simulink model "correct_sm_circle (1)"  (R2022b)
settings: Solver=VariableStepAuto  StartTime=0.0  StopTime=25  RelTol=1e-3
values from neighbouring files (symbols this model uses):
  Fxg = 0.005    [constants (3).m]
  Fyg = 0.005    [constants (3).m]
  g = 9.81    [constants (3).m]
  Ixx = 2.3951 * 10^-5    (= 2.3951e-05)    [constants (3).m]
  Iyy = 2.3951 * 10^-5    (= 2.3951e-05)    [constants (3).m]
  Izz = 3.2347 * 10^-5    (= 3.2347e-05)    [constants (3).m]
  kf = 0.005022    [constants (3).m]
  km = 1.858*10^-5    (= 1.858e-05)    [constants (3).m]
  L = 32 * 10^-3    (= 0.032)    [constants (3).m]
  m = 0.034    [constants (3).m]
libraries: slpidlib x6, matrix_library x1, aerolibutil x1
settings Model: Creator=nayan  LastModifiedBy=Sreejeet Maity
settings SolverCC: ZeroCrossAlgorithm=Adaptive
settings DebuggingCC: IgnoredZcDiagnostic=none
settings ModelReferenceCC: EnableRefExpFcnMdlSchedulingChecks=on

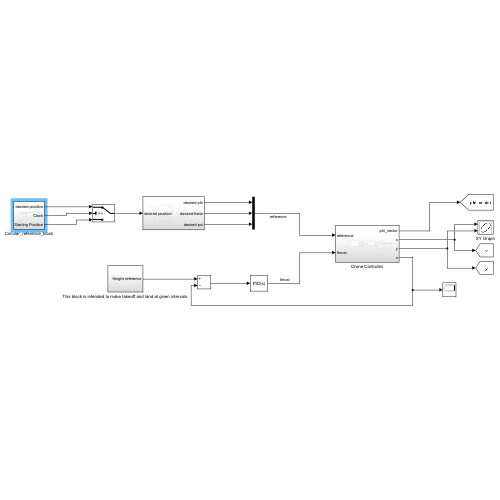
[thumbnail: Simulink's stored preview of the top-level diagram]
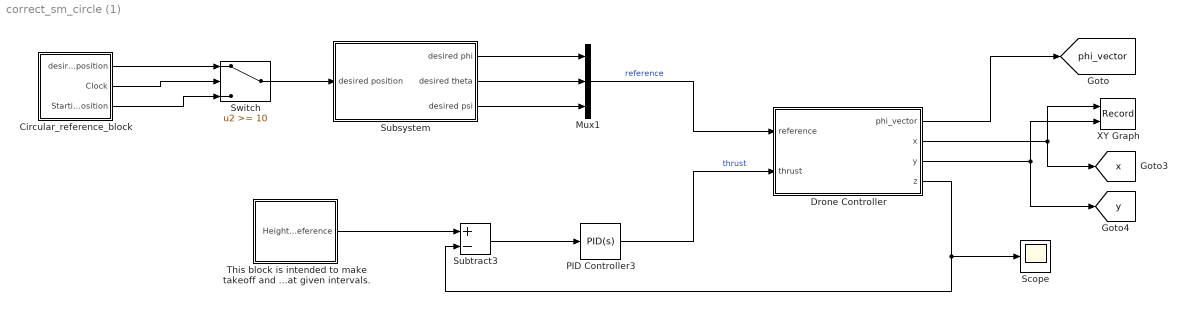
== system correct_sm_circle (1) ==
  Circular_reference_block : Subsystem
  Drone Controller : Subsystem
  Mux1 : Mux  Inputs=3
  PID Controller3 : slpidlib/PID Controller  Controller=PID  Form=Parallel  TimeDomain=Continuous-time  UseExternalTs=off  SampleTime=-1  IntegratorMethod=Forward Euler  FilterMethod=Forward Euler  ControllerParametersSource=internal  P=291  I=47.33  UseKiTs=off  D=18.69  N=1478  UseFilter=on  TunerSelectOption=Transfer Function Based (PID Tuner App)  InitialConditionSource=internal  InitialConditionForIntegrator=0  InitialConditionForFilter=0  DifferentiatorICPrevScaledInput=0  ExternalReset=none  TrackingMode=off  Kt=1  LimitOutput=off  SatLimitsSource=internal  UpperSaturationLimit=inf  LowerSaturationLimit=-inf  LinearizeAsGain=on  AntiWindupMode=none  Kb=1  LimitIntegrator=off  UpperIntegratorSaturationLimit=inf  LowerIntegratorSaturationLimit=-inf  POutMin=[]  POutMax=[]  IOutMin=[]  IOutMax=[]  DOutMin=[]  DOutMax=[]  NOutMin=[]  NOutMax=[]  SumOutMin=[]  SumOutMax=[]  SaturationOutMin=[]  SaturationOutMax=[]  PParamMin=[]  PParamMax=[]  IParamMin=[]  IParamMax=[]  DParamMin=[]  DParamMax=[]  NParamMin=[]  NParamMax=[]  KbParamMin=[]  KbParamMax=[]  KtParamMin=[]  KtParamMax=[]  KbOutMin=[]  KbOutMax=[]  KtOutMin=[]  KtOutMax=[]  IntegratorOutMin=[]  IntegratorOutMax=[]  FilterOutMin=[]  FilterOutMax=[]  SumI1OutMin=[]  SumI1OutMax=[]  SumI2OutMin=[]  SumI2OutMax=[]  SumI3OutMin=[]  SumI3OutMax=[]  SumI4OutMin=[]  SumI4OutMax=[]  SumDOutMin=[]  SumDOutMax=[]  DifferentiatorOutMin=[]  DifferentiatorOutMax=[]  FilterDiffOutCoefMin=[]  FilterDiffOutCoefMax=[]  ReciprocalOutMin=[]  ReciprocalOutMax=[]  SumDenOutMin=[]  SumDenOutMax=[]  SumNumOutMin=[]  SumNumOutMax=[]  DivideOutMin=[]  DivideOutMax=[]  UdiffTsProdOutMin=[]  UdiffTsProdOutMax=[]  NTsProdOutMin=[]  NTsProdOutMax=[]  UintegralTsProdOutMin=[]  UintegralTsProdOutMax=[]  UngainTsProdOutMin=[]  UngainTsProdOutMax=[]  ClampingZeroOutDataTypeStr=Inherit: Inherit via back propagation  ClampingZeroOutMin=[]  ClampingZeroOutMax=[]  FilterDenConstantOutDataTypeStr=Inherit: Inherit via back propagation  FilterDenConstantOutMin=[]  FilterDenConstantOutMax=[]  PCopyOutDataTypeStr=Inherit: Inherit via back propagation  PCopyOutMin=[]  PCopyOutMax=[]  NCopyOutDataTypeStr=Inherit: Inherit via back propagation  NCopyOutMin=[]  NCopyOutMax=[]  IntegratorContinuousStateAttributes=''  IntegratorStateMustResolveToSignalObject=off  IntegratorRTWStateStorageClass=Auto  FilterContinuousStateAttributes=''  FilterStateMustResolveToSignalObject=off  FilterRTWStateStorageClass=Auto  ParallelPVariant=InternalParameters  IdealPVariant=Disabled  IVariant=InternalParameters  DVariant=InternalParameters  IntegratorVariant=Continuous  SatVariant=Disabled  AWVariant=Passthrough  PCopyVariant=Disabled  TRVariant=Disabled  FdbkBlocksVariant=Forward  IdealPFdbkVariant=Disabled  SatFdbkVariant=Disabled  DerivativeFilterVariant=ContFilter  NVariant=InternalParameters  NCopyVariant=Disabled  FilterICVariant=InternalICsFilter  IntegratorICVariant=InternalICs  ExternalResetVariant=Disabled  TRSumVariant=Passthrough  SumFdbkVariant=Disabled  SumVariant=Sum_PID  TsampFilterVariant=InternalTs  TsampNgainVariant=Passthrough  TsampIntegralVariant=Passthrough  ExternalSaturationOutDataTypeStr=Inherit: Same as second input
  Scope : Scope
  Subsystem : Subsystem
  Subtract3 : Sum  Inputs=+-
  Switch : Switch  Threshold=10  SaturateOnIntegerOverflow=off  InputSameDT=off
  This block is intended to make takeoff and land at given intervals. : Subsystem
  XY Graph : Record  FileSettingsInternal="{\"entries\":[{\"content\":{\"excelSettings\":{\"content\":{},\"type\":\"Streamout.ExcelSettings\"}},\"type\":\"Streamout.FileSettingStorage\",\"uuid\":\"8c642e62-005c-4423-a761-cbdb6bbecf0f\"}],\"packageUris\":[\"http://schema.mathworks.com/mf0/streamout_blocks/R2020a\"],\"version\":\"1.0\"}"  Layout=[1 1]  SignalsInternal="{\"entries\":[{\"content\":{\"signals\":[{\"content\":{\"blockPath\":[\"correct_sm_circle/XY Graph\"],\"channel\":[],\"dimensions\":[1],\"domain\":\"correct_sm_circle/XY Graph\",\"lineColor\":\"#a2142f\",\"plots\":[1],\"port\":1,\"sid\":[\"\"],\"signalID\":12972,\"signalName\":\"Drone Controller:2\"},\"type\":\"RecordBlkView.Signal\",\"uuid\":\"ff125678-109d-4bf1-ad2c-892bd237ab7f\"},{\"content\":{\"blockPath\":[\"correct_sm_circle/XY Graph\"],\"channel\":[],\"dimensions\":[1],\"domain\":\"correct_sm_circle/XY Graph\",\"lineColor\":\"#139fff\",\"plots\":[1],\"port\":2,\"sid\":[\"\"],\"signalID\":12976,\"signalName\":\"Drone Controller:3\"},\"type\":\"RecordBlkView.Signal\",\"uuid\":\"d1c5deef-ede5-4cd3-9f15-060bb912ac46\"}]},\"type\":\"RecordBlkView.InputSignals\",\"uuid\":\"1252a0e8-627c-4691-9929-d6fd4d200b48\"}],\"packageUris\":[\"http://schema.mathworks.com/mf0/streamout_blocks/R2020a\"],\"version\":\"1.0\"}"  VisualizationBindings="{\"xyplotplugin\":{\"info\":[{\"series\":[{\"bindingParametersList\":[{\"parameter\":\"X-Axis\",\"signalID\":12972,\"signalName\":\"Drone Controller:2\"},{\"parameter\":\"Y-Axis\",\"signalID\":12976,\"signalName\":\"Drone Controller:3\"}],\"seriesID\":36752}],\"subplotID\":1}]}}"  CompatibilityTag=XY
  tag scope: phi_vector=global, x=global, y=global
  wires:
  Subtract3/1 -> PID Controller3/1
  Subsystem/1(desired phi) -> Mux1/1
  Subsystem/2(desired theta) -> Mux1/2
  Subsystem/3(desired psi) -> Mux1/3
  Switch/1 -> Subsystem/1(desired position)
  Circular_reference_block/1(desired position) -> Switch/1
  Circular_reference_block/2(Clock) -> Switch/2
  Circular_reference_block/3(Starting Position) -> Switch/3
  This block is intended to make takeoff and land at given intervals./1(Height reference) -> Subtract3/1
  Drone Controller/2(x) -> XY Graph/1, [x]
  Drone Controller/3(y) -> XY Graph/2, [y]
  Drone Controller/4(z) -> Subtract3/2, Scope/1
  Mux1/1 -> Drone Controller/1(reference)  "reference"
  PID Controller3/1 -> Drone Controller/2(thrust)  "thrust"
  Drone Controller/1(phi_vector) -> [phi_vector]

== system correct_sm_circle (1)/Circular_reference_block ==
  Circular_reference : Subsystem
  Desired Position : Scope
  Initial Position : Constant  Value=[1 ; 0]
  Mux3 : Mux  Inputs=2
  desired position : Outport
  Clock : Outport  Port=2
  Starting Position : Outport  Port=3
  wires:
  Initial Position/1 -> Starting Position/1
  Mux3/1 -> desired position/1, Desired Position/1  "desired position"
  Circular_reference/2(cos(t-10)) -> Mux3/1
  Circular_reference/3(sin(t-10)) -> Mux3/2
  Circular_reference/1(Clock) -> Clock/1

== system correct_sm_circle (1)/Drone Controller ==
  reference : Inport
  thrust : Inport  Port=2
  Attitude Controller : Subsystem
  Drone_1 : Subsystem
  Mux : Mux
  phi_vector : Outport
  x : Outport  Port=2
  y : Outport  Port=3
  z : Outport  Port=4
  wires:
  Drone_1/4(z) -> z/1
  Attitude Controller/1(w1_square) -> Mux/1
  Attitude Controller/3(w3_square) -> Mux/3
  Drone_1/2(x) -> x/1
  Mux/1 -> Drone_1/1(squares of motor omega in rpm)  "squares of motor omega in rpm"
  Drone_1/3(y) -> y/1
  Attitude Controller/2(w2_square) -> Mux/2
  Attitude Controller/4(w4_square) -> Mux/4
  Drone_1/1(phi_vector) -> phi_vector/1
  thrust/1 -> Attitude Controller/2("thrust ")
  reference/1 -> Attitude Controller/1(roll pitch yaw reference)

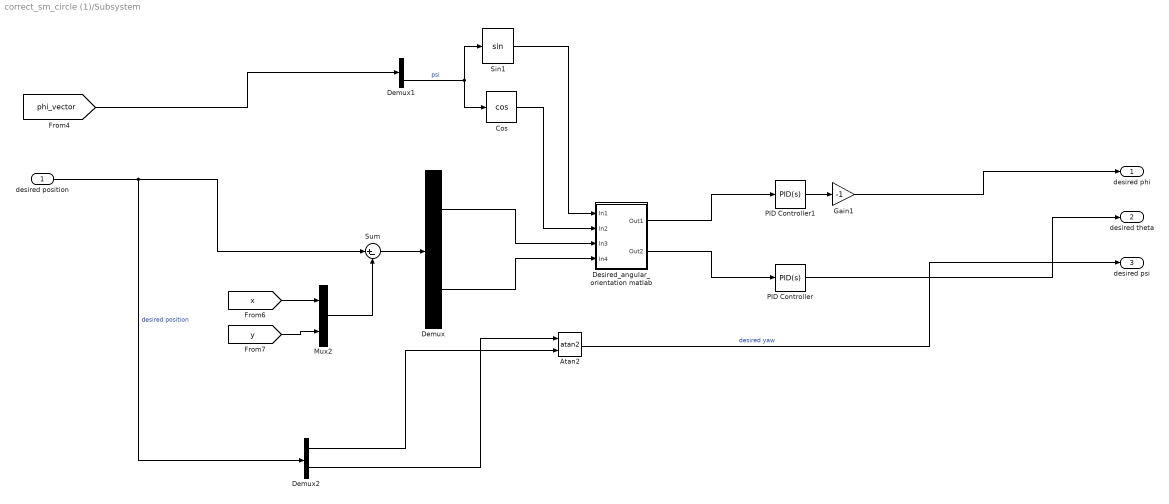
== system correct_sm_circle (1)/Subsystem ==
  desired position : Inport
  Atan2 : Trigonometry  Operator=atan2
  Cos : Trigonometry  Operator=cos
  Demux : Demux  Outputs=2
  Demux1 : Demux  Outputs=3
  Demux2 : Demux  Outputs=2
  Desired_angular_orientation matlab : Subsystem
  Gain1 : Gain  Gain=-1
  Mux2 : Mux  Inputs=2
  PID Controller : slpidlib/PID Controller  Controller=PID  Form=Parallel  TimeDomain=Continuous-time  UseExternalTs=off  SampleTime=-1  IntegratorMethod=Forward Euler  FilterMethod=Forward Euler  ControllerParametersSource=internal  P=0.43  I=0.043  UseKiTs=off  D=0.042  N=10000  UseFilter=on  TunerSelectOption=Transfer Function Based (PID Tuner App)  InitialConditionSource=internal  InitialConditionForIntegrator=0  InitialConditionForFilter=0  DifferentiatorICPrevScaledInput=0  ExternalReset=none  TrackingMode=off  Kt=1  LimitOutput=off  SatLimitsSource=internal  UpperSaturationLimit=inf  LowerSaturationLimit=-inf  LinearizeAsGain=on  AntiWindupMode=none  Kb=1  LimitIntegrator=off  UpperIntegratorSaturationLimit=inf  LowerIntegratorSaturationLimit=-inf  POutMin=[]  POutMax=[]  IOutMin=[]  IOutMax=[]  DOutMin=[]  DOutMax=[]  NOutMin=[]  NOutMax=[]  SumOutMin=[]  SumOutMax=[]  SaturationOutMin=[]  SaturationOutMax=[]  PParamMin=[]  PParamMax=[]  IParamMin=[]  IParamMax=[]  DParamMin=[]  DParamMax=[]  NParamMin=[]  NParamMax=[]  KbParamMin=[]  KbParamMax=[]  KtParamMin=[]  KtParamMax=[]  KbOutMin=[]  KbOutMax=[]  KtOutMin=[]  KtOutMax=[]  IntegratorOutMin=[]  IntegratorOutMax=[]  FilterOutMin=[]  FilterOutMax=[]  SumI1OutMin=[]  SumI1OutMax=[]  SumI2OutMin=[]  SumI2OutMax=[]  SumI3OutMin=[]  SumI3OutMax=[]  SumI4OutMin=[]  SumI4OutMax=[]  SumDOutMin=[]  SumDOutMax=[]  DifferentiatorOutMin=[]  DifferentiatorOutMax=[]  FilterDiffOutCoefMin=[]  FilterDiffOutCoefMax=[]  ReciprocalOutMin=[]  ReciprocalOutMax=[]  SumDenOutMin=[]  SumDenOutMax=[]  SumNumOutMin=[]  SumNumOutMax=[]  DivideOutMin=[]  DivideOutMax=[]  UdiffTsProdOutMin=[]  UdiffTsProdOutMax=[]  NTsProdOutMin=[]  NTsProdOutMax=[]  UintegralTsProdOutMin=[]  UintegralTsProdOutMax=[]  UngainTsProdOutMin=[]  UngainTsProdOutMax=[]  ClampingZeroOutDataTypeStr=Inherit: Inherit via back propagation  ClampingZeroOutMin=[]  ClampingZeroOutMax=[]  FilterDenConstantOutDataTypeStr=Inherit: Inherit via back propagation  FilterDenConstantOutMin=[]  FilterDenConstantOutMax=[]  PCopyOutDataTypeStr=Inherit: Inherit via back propagation  PCopyOutMin=[]  PCopyOutMax=[]  NCopyOutDataTypeStr=Inherit: Inherit via back propagation  NCopyOutMin=[]  NCopyOutMax=[]  IntegratorContinuousStateAttributes=''  IntegratorStateMustResolveToSignalObject=off  IntegratorRTWStateStorageClass=Auto  FilterContinuousStateAttributes=''  FilterStateMustResolveToSignalObject=off  FilterRTWStateStorageClass=Auto  ParallelPVariant=InternalParameters  IdealPVariant=Disabled  IVariant=InternalParameters  DVariant=InternalParameters  IntegratorVariant=Continuous  SatVariant=Disabled  AWVariant=Passthrough  PCopyVariant=Disabled  TRVariant=Disabled  FdbkBlocksVariant=Forward  IdealPFdbkVariant=Disabled  SatFdbkVariant=Disabled  DerivativeFilterVariant=ContFilter  NVariant=InternalParameters  NCopyVariant=Disabled  FilterICVariant=InternalICsFilter  IntegratorICVariant=InternalICs  ExternalResetVariant=Disabled  TRSumVariant=Passthrough  SumFdbkVariant=Disabled  SumVariant=Sum_PID  TsampFilterVariant=InternalTs  TsampNgainVariant=Passthrough  TsampIntegralVariant=Passthrough  ExternalSaturationOutDataTypeStr=Inherit: Same as second input
  PID Controller1 : slpidlib/PID Controller  Controller=PID  Form=Parallel  TimeDomain=Continuous-time  UseExternalTs=off  SampleTime=-1  IntegratorMethod=Forward Euler  FilterMethod=Forward Euler  ControllerParametersSource=internal  P=0.43  I=0.0412  UseKiTs=off  D=0.043  N=10000  UseFilter=on  TunerSelectOption=Transfer Function Based (PID Tuner App)  InitialConditionSource=internal  InitialConditionForIntegrator=0  InitialConditionForFilter=0  DifferentiatorICPrevScaledInput=0  ExternalReset=none  TrackingMode=off  Kt=1  LimitOutput=off  SatLimitsSource=internal  UpperSaturationLimit=inf  LowerSaturationLimit=-inf  LinearizeAsGain=on  AntiWindupMode=none  Kb=1  LimitIntegrator=off  UpperIntegratorSaturationLimit=inf  LowerIntegratorSaturationLimit=-inf  POutMin=[]  POutMax=[]  IOutMin=[]  IOutMax=[]  DOutMin=[]  DOutMax=[]  NOutMin=[]  NOutMax=[]  SumOutMin=[]  SumOutMax=[]  SaturationOutMin=[]  SaturationOutMax=[]  PParamMin=[]  PParamMax=[]  IParamMin=[]  IParamMax=[]  DParamMin=[]  DParamMax=[]  NParamMin=[]  NParamMax=[]  KbParamMin=[]  KbParamMax=[]  KtParamMin=[]  KtParamMax=[]  KbOutMin=[]  KbOutMax=[]  KtOutMin=[]  KtOutMax=[]  IntegratorOutMin=[]  IntegratorOutMax=[]  FilterOutMin=[]  FilterOutMax=[]  SumI1OutMin=[]  SumI1OutMax=[]  SumI2OutMin=[]  SumI2OutMax=[]  SumI3OutMin=[]  SumI3OutMax=[]  SumI4OutMin=[]  SumI4OutMax=[]  SumDOutMin=[]  SumDOutMax=[]  DifferentiatorOutMin=[]  DifferentiatorOutMax=[]  FilterDiffOutCoefMin=[]  FilterDiffOutCoefMax=[]  ReciprocalOutMin=[]  ReciprocalOutMax=[]  SumDenOutMin=[]  SumDenOutMax=[]  SumNumOutMin=[]  SumNumOutMax=[]  DivideOutMin=[]  DivideOutMax=[]  UdiffTsProdOutMin=[]  UdiffTsProdOutMax=[]  NTsProdOutMin=[]  NTsProdOutMax=[]  UintegralTsProdOutMin=[]  UintegralTsProdOutMax=[]  UngainTsProdOutMin=[]  UngainTsProdOutMax=[]  ClampingZeroOutDataTypeStr=Inherit: Inherit via back propagation  ClampingZeroOutMin=[]  ClampingZeroOutMax=[]  FilterDenConstantOutDataTypeStr=Inherit: Inherit via back propagation  FilterDenConstantOutMin=[]  FilterDenConstantOutMax=[]  PCopyOutDataTypeStr=Inherit: Inherit via back propagation  PCopyOutMin=[]  PCopyOutMax=[]  NCopyOutDataTypeStr=Inherit: Inherit via back propagation  NCopyOutMin=[]  NCopyOutMax=[]  IntegratorContinuousStateAttributes=''  IntegratorStateMustResolveToSignalObject=off  IntegratorRTWStateStorageClass=Auto  FilterContinuousStateAttributes=''  FilterStateMustResolveToSignalObject=off  FilterRTWStateStorageClass=Auto  ParallelPVariant=InternalParameters  IdealPVariant=Disabled  IVariant=InternalParameters  DVariant=InternalParameters  IntegratorVariant=Continuous  SatVariant=Disabled  AWVariant=Passthrough  PCopyVariant=Disabled  TRVariant=Disabled  FdbkBlocksVariant=Forward  IdealPFdbkVariant=Disabled  SatFdbkVariant=Disabled  DerivativeFilterVariant=ContFilter  NVariant=InternalParameters  NCopyVariant=Disabled  FilterICVariant=InternalICsFilter  IntegratorICVariant=InternalICs  ExternalResetVariant=Disabled  TRSumVariant=Passthrough  SumFdbkVariant=Disabled  SumVariant=Sum_PID  TsampFilterVariant=InternalTs  TsampNgainVariant=Passthrough  TsampIntegralVariant=Passthrough  ExternalSaturationOutDataTypeStr=Inherit: Same as second input
  Sin1 : Trigonometry
  Sum : Sum  Inputs=|+-
  desired phi : Outport
  desired theta : Outport  Port=2
  desired psi : Outport  Port=3
  wires:
  Sum/1 -> Demux/1
  PID Controller/1 -> desired theta/1
  PID Controller1/1 -> Gain1/1
  Gain1/1 -> desired phi/1
  Demux1/3 -> Cos/1, Sin1/1  "psi"
  [x] -> Mux2/1
  Mux2/1 -> Sum/2
  [y] -> Mux2/2
  [phi_vector] -> Demux1/1
  desired position/1 -> Demux2/1, Sum/1  "desired position"
  Atan2/1 -> desired psi/1  "desired yaw"
  Demux2/2 -> Atan2/1
  Demux2/1 -> Atan2/2
  Sin1/1 -> Desired_angular_orientation matlab/1(In1)
  Cos/1 -> Desired_angular_orientation matlab/2(In2)
  Demux/1 -> Desired_angular_orientation matlab/3(In3)
  Demux/2 -> Desired_angular_orientation matlab/4(In4)
  Desired_angular_orientation matlab/1(Out1) -> PID Controller1/1
  Desired_angular_orientation matlab/2(Out2) -> PID Controller/1

== system correct_sm_circle (1)/This block is intended to make takeoff and land at given intervals. ==
  Clock : Clock
  Constant : Constant
  Constant3 : Constant  Value=0
  Switch1 : Switch  Threshold=20  SaturateOnIntegerOverflow=off  InputSameDT=off
  Height reference : Outport
  wires:
  Clock/1 -> Switch1/2
  Constant/1 -> Switch1/3  "Height reference"
  Constant3/1 -> Switch1/1  "Height reference"
  Switch1/1 -> Height reference/1  "Height reference"

== system correct_sm_circle (1)/Circular_reference_block/Circular_reference ==
  Clock1 : Clock
  Cos : Trigonometry  Operator=cos
  Sin1 : Trigonometry
  Subtract : Sum  Inputs=+-
  time to take_off : Constant  Value=10
  Clock : Outport
  cos(t-10) : Outport  Port=2
  sin(t-10) : Outport  Port=3
  wires:
  Subtract/1 -> Cos/1, Sin1/1
  Clock1/1 -> Clock/1, Subtract/1
  Cos/1 -> cos(t-10)/1
  time to take_off/1 -> Subtract/2
  Sin1/1 -> sin(t-10)/1

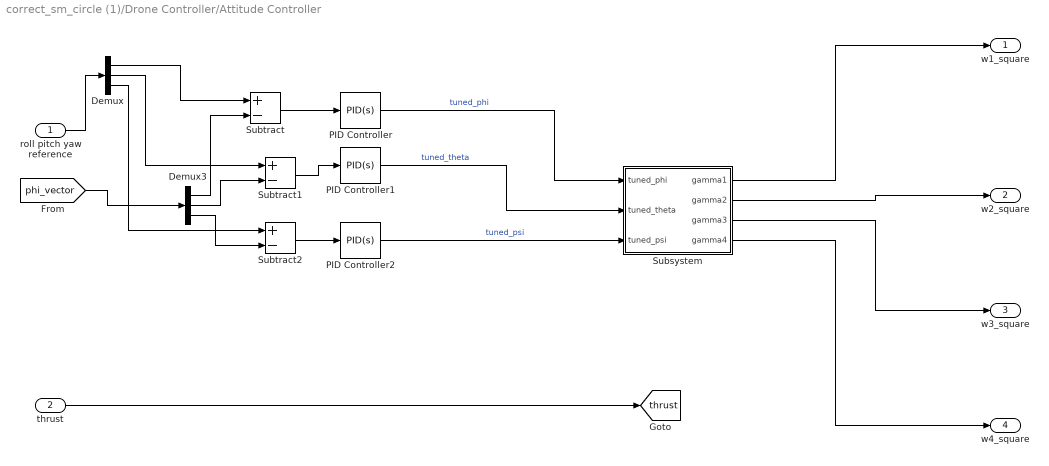
== system correct_sm_circle (1)/Drone Controller/Attitude Controller ==
  roll pitch yaw reference : Inport
  "thrust " : Inport  Port=2
  Demux : Demux  Outputs=3
  Demux3 : Demux  Outputs=3
  PID Controller : slpidlib/PID Controller  Controller=PID  Form=Parallel  TimeDomain=Continuous-time  UseExternalTs=off  SampleTime=-1  IntegratorMethod=Forward Euler  FilterMethod=Forward Euler  ControllerParametersSource=internal  P=96.35  I=143.26  UseKiTs=off  D=23.32  N=10000  UseFilter=on  TunerSelectOption=Transfer Function Based (PID Tuner App)  InitialConditionSource=internal  InitialConditionForIntegrator=0  InitialConditionForFilter=0  DifferentiatorICPrevScaledInput=0  ExternalReset=none  TrackingMode=off  Kt=1  LimitOutput=off  SatLimitsSource=internal  UpperSaturationLimit=inf  LowerSaturationLimit=-inf  LinearizeAsGain=on  AntiWindupMode=none  Kb=1  LimitIntegrator=off  UpperIntegratorSaturationLimit=inf  LowerIntegratorSaturationLimit=-inf  POutMin=[]  POutMax=[]  IOutMin=[]  IOutMax=[]  DOutMin=[]  DOutMax=[]  NOutMin=[]  NOutMax=[]  SumOutMin=[]  SumOutMax=[]  SaturationOutMin=[]  SaturationOutMax=[]  PParamMin=[]  PParamMax=[]  IParamMin=[]  IParamMax=[]  DParamMin=[]  DParamMax=[]  NParamMin=[]  NParamMax=[]  KbParamMin=[]  KbParamMax=[]  KtParamMin=[]  KtParamMax=[]  KbOutMin=[]  KbOutMax=[]  KtOutMin=[]  KtOutMax=[]  IntegratorOutMin=[]  IntegratorOutMax=[]  FilterOutMin=[]  FilterOutMax=[]  SumI1OutMin=[]  SumI1OutMax=[]  SumI2OutMin=[]  SumI2OutMax=[]  SumI3OutMin=[]  SumI3OutMax=[]  SumI4OutMin=[]  SumI4OutMax=[]  SumDOutMin=[]  SumDOutMax=[]  DifferentiatorOutMin=[]  DifferentiatorOutMax=[]  FilterDiffOutCoefMin=[]  FilterDiffOutCoefMax=[]  ReciprocalOutMin=[]  ReciprocalOutMax=[]  SumDenOutMin=[]  SumDenOutMax=[]  SumNumOutMin=[]  SumNumOutMax=[]  DivideOutMin=[]  DivideOutMax=[]  UdiffTsProdOutMin=[]  UdiffTsProdOutMax=[]  NTsProdOutMin=[]  NTsProdOutMax=[]  UintegralTsProdOutMin=[]  UintegralTsProdOutMax=[]  UngainTsProdOutMin=[]  UngainTsProdOutMax=[]  ClampingZeroOutDataTypeStr=Inherit: Inherit via back propagation  ClampingZeroOutMin=[]  ClampingZeroOutMax=[]  FilterDenConstantOutDataTypeStr=Inherit: Inherit via back propagation  FilterDenConstantOutMin=[]  FilterDenConstantOutMax=[]  PCopyOutDataTypeStr=Inherit: Inherit via back propagation  PCopyOutMin=[]  PCopyOutMax=[]  NCopyOutDataTypeStr=Inherit: Inherit via back propagation  NCopyOutMin=[]  NCopyOutMax=[]  IntegratorContinuousStateAttributes=''  IntegratorStateMustResolveToSignalObject=off  IntegratorRTWStateStorageClass=Auto  FilterContinuousStateAttributes=''  FilterStateMustResolveToSignalObject=off  FilterRTWStateStorageClass=Auto  ParallelPVariant=InternalParameters  IdealPVariant=Disabled  IVariant=InternalParameters  DVariant=InternalParameters  IntegratorVariant=Continuous  SatVariant=Disabled  AWVariant=Passthrough  PCopyVariant=Disabled  TRVariant=Disabled  FdbkBlocksVariant=Forward  IdealPFdbkVariant=Disabled  SatFdbkVariant=Disabled  DerivativeFilterVariant=ContFilter  NVariant=InternalParameters  NCopyVariant=Disabled  FilterICVariant=InternalICsFilter  IntegratorICVariant=InternalICs  ExternalResetVariant=Disabled  TRSumVariant=Passthrough  SumFdbkVariant=Disabled  SumVariant=Sum_PID  TsampFilterVariant=InternalTs  TsampNgainVariant=Passthrough  TsampIntegralVariant=Passthrough  ExternalSaturationOutDataTypeStr=Inherit: Same as second input
  PID Controller1 : slpidlib/PID Controller  Controller=PID  Form=Parallel  TimeDomain=Continuous-time  UseExternalTs=off  SampleTime=-1  IntegratorMethod=Forward Euler  FilterMethod=Forward Euler  ControllerParametersSource=internal  P=96.36  I=143.5  UseKiTs=off  D=22.32  N=10000  UseFilter=on  TunerSelectOption=Transfer Function Based (PID Tuner App)  InitialConditionSource=internal  InitialConditionForIntegrator=0  InitialConditionForFilter=0  DifferentiatorICPrevScaledInput=0  ExternalReset=none  TrackingMode=off  Kt=1  LimitOutput=off  SatLimitsSource=internal  UpperSaturationLimit=inf  LowerSaturationLimit=-inf  LinearizeAsGain=on  AntiWindupMode=none  Kb=1  LimitIntegrator=off  UpperIntegratorSaturationLimit=inf  LowerIntegratorSaturationLimit=-inf  POutMin=[]  POutMax=[]  IOutMin=[]  IOutMax=[]  DOutMin=[]  DOutMax=[]  NOutMin=[]  NOutMax=[]  SumOutMin=[]  SumOutMax=[]  SaturationOutMin=[]  SaturationOutMax=[]  PParamMin=[]  PParamMax=[]  IParamMin=[]  IParamMax=[]  DParamMin=[]  DParamMax=[]  NParamMin=[]  NParamMax=[]  KbParamMin=[]  KbParamMax=[]  KtParamMin=[]  KtParamMax=[]  KbOutMin=[]  KbOutMax=[]  KtOutMin=[]  KtOutMax=[]  IntegratorOutMin=[]  IntegratorOutMax=[]  FilterOutMin=[]  FilterOutMax=[]  SumI1OutMin=[]  SumI1OutMax=[]  SumI2OutMin=[]  SumI2OutMax=[]  SumI3OutMin=[]  SumI3OutMax=[]  SumI4OutMin=[]  SumI4OutMax=[]  SumDOutMin=[]  SumDOutMax=[]  DifferentiatorOutMin=[]  DifferentiatorOutMax=[]  FilterDiffOutCoefMin=[]  FilterDiffOutCoefMax=[]  ReciprocalOutMin=[]  ReciprocalOutMax=[]  SumDenOutMin=[]  SumDenOutMax=[]  SumNumOutMin=[]  SumNumOutMax=[]  DivideOutMin=[]  DivideOutMax=[]  UdiffTsProdOutMin=[]  UdiffTsProdOutMax=[]  NTsProdOutMin=[]  NTsProdOutMax=[]  UintegralTsProdOutMin=[]  UintegralTsProdOutMax=[]  UngainTsProdOutMin=[]  UngainTsProdOutMax=[]  ClampingZeroOutDataTypeStr=Inherit: Inherit via back propagation  ClampingZeroOutMin=[]  ClampingZeroOutMax=[]  FilterDenConstantOutDataTypeStr=Inherit: Inherit via back propagation  FilterDenConstantOutMin=[]  FilterDenConstantOutMax=[]  PCopyOutDataTypeStr=Inherit: Inherit via back propagation  PCopyOutMin=[]  PCopyOutMax=[]  NCopyOutDataTypeStr=Inherit: Inherit via back propagation  NCopyOutMin=[]  NCopyOutMax=[]  IntegratorContinuousStateAttributes=''  IntegratorStateMustResolveToSignalObject=off  IntegratorRTWStateStorageClass=Auto  FilterContinuousStateAttributes=''  FilterStateMustResolveToSignalObject=off  FilterRTWStateStorageClass=Auto  ParallelPVariant=InternalParameters  IdealPVariant=Disabled  IVariant=InternalParameters  DVariant=InternalParameters  IntegratorVariant=Continuous  SatVariant=Disabled  AWVariant=Passthrough  PCopyVariant=Disabled  TRVariant=Disabled  FdbkBlocksVariant=Forward  IdealPFdbkVariant=Disabled  SatFdbkVariant=Disabled  DerivativeFilterVariant=ContFilter  NVariant=InternalParameters  NCopyVariant=Disabled  FilterICVariant=InternalICsFilter  IntegratorICVariant=InternalICs  ExternalResetVariant=Disabled  TRSumVariant=Passthrough  SumFdbkVariant=Disabled  SumVariant=Sum_PID  TsampFilterVariant=InternalTs  TsampNgainVariant=Passthrough  TsampIntegralVariant=Passthrough  ExternalSaturationOutDataTypeStr=Inherit: Same as second input
  PID Controller2 : slpidlib/PID Controller  Controller=PID  Form=Parallel  TimeDomain=Continuous-time  UseExternalTs=off  SampleTime=-1  IntegratorMethod=Forward Euler  FilterMethod=Forward Euler  ControllerParametersSource=internal  P=96.36  I=146.25  UseKiTs=off  D=22.37  N=10000  UseFilter=on  TunerSelectOption=Transfer Function Based (PID Tuner App)  InitialConditionSource=internal  InitialConditionForIntegrator=0  InitialConditionForFilter=0  DifferentiatorICPrevScaledInput=0  ExternalReset=none  TrackingMode=off  Kt=1  LimitOutput=off  SatLimitsSource=internal  UpperSaturationLimit=inf  LowerSaturationLimit=-inf  LinearizeAsGain=on  AntiWindupMode=none  Kb=1  LimitIntegrator=off  UpperIntegratorSaturationLimit=inf  LowerIntegratorSaturationLimit=-inf  POutMin=[]  POutMax=[]  IOutMin=[]  IOutMax=[]  DOutMin=[]  DOutMax=[]  NOutMin=[]  NOutMax=[]  SumOutMin=[]  SumOutMax=[]  SaturationOutMin=[]  SaturationOutMax=[]  PParamMin=[]  PParamMax=[]  IParamMin=[]  IParamMax=[]  DParamMin=[]  DParamMax=[]  NParamMin=[]  NParamMax=[]  KbParamMin=[]  KbParamMax=[]  KtParamMin=[]  KtParamMax=[]  KbOutMin=[]  KbOutMax=[]  KtOutMin=[]  KtOutMax=[]  IntegratorOutMin=[]  IntegratorOutMax=[]  FilterOutMin=[]  FilterOutMax=[]  SumI1OutMin=[]  SumI1OutMax=[]  SumI2OutMin=[]  SumI2OutMax=[]  SumI3OutMin=[]  SumI3OutMax=[]  SumI4OutMin=[]  SumI4OutMax=[]  SumDOutMin=[]  SumDOutMax=[]  DifferentiatorOutMin=[]  DifferentiatorOutMax=[]  FilterDiffOutCoefMin=[]  FilterDiffOutCoefMax=[]  ReciprocalOutMin=[]  ReciprocalOutMax=[]  SumDenOutMin=[]  SumDenOutMax=[]  SumNumOutMin=[]  SumNumOutMax=[]  DivideOutMin=[]  DivideOutMax=[]  UdiffTsProdOutMin=[]  UdiffTsProdOutMax=[]  NTsProdOutMin=[]  NTsProdOutMax=[]  UintegralTsProdOutMin=[]  UintegralTsProdOutMax=[]  UngainTsProdOutMin=[]  UngainTsProdOutMax=[]  ClampingZeroOutDataTypeStr=Inherit: Inherit via back propagation  ClampingZeroOutMin=[]  ClampingZeroOutMax=[]  FilterDenConstantOutDataTypeStr=Inherit: Inherit via back propagation  FilterDenConstantOutMin=[]  FilterDenConstantOutMax=[]  PCopyOutDataTypeStr=Inherit: Inherit via back propagation  PCopyOutMin=[]  PCopyOutMax=[]  NCopyOutDataTypeStr=Inherit: Inherit via back propagation  NCopyOutMin=[]  NCopyOutMax=[]  IntegratorContinuousStateAttributes=''  IntegratorStateMustResolveToSignalObject=off  IntegratorRTWStateStorageClass=Auto  FilterContinuousStateAttributes=''  FilterStateMustResolveToSignalObject=off  FilterRTWStateStorageClass=Auto  ParallelPVariant=InternalParameters  IdealPVariant=Disabled  IVariant=InternalParameters  DVariant=InternalParameters  IntegratorVariant=Continuous  SatVariant=Disabled  AWVariant=Passthrough  PCopyVariant=Disabled  TRVariant=Disabled  FdbkBlocksVariant=Forward  IdealPFdbkVariant=Disabled  SatFdbkVariant=Disabled  DerivativeFilterVariant=ContFilter  NVariant=InternalParameters  NCopyVariant=Disabled  FilterICVariant=InternalICsFilter  IntegratorICVariant=InternalICs  ExternalResetVariant=Disabled  TRSumVariant=Passthrough  SumFdbkVariant=Disabled  SumVariant=Sum_PID  TsampFilterVariant=InternalTs  TsampNgainVariant=Passthrough  TsampIntegralVariant=Passthrough  ExternalSaturationOutDataTypeStr=Inherit: Same as second input
  Subsystem : Subsystem
  Subtract : Sum  Inputs=+-
  Subtract1 : Sum  Inputs=+-
  Subtract2 : Sum  Inputs=+-
  w1_square : Outport
  w2_square : Outport  Port=2
  w3_square : Outport  Port=3
  w4_square : Outport  Port=4
  tag scope: thrust=global
  wires:
  Subtract2/1 -> PID Controller2/1
  Demux3/2 -> Subtract1/2
  [phi_vector] -> Demux3/1
  Demux3/3 -> Subtract2/2
  Subtract1/1 -> PID Controller1/1
  Subtract/1 -> PID Controller/1
  Demux3/1 -> Subtract/2
  roll pitch yaw reference/1 -> Demux/1
  Demux/1 -> Subtract/1
  Demux/2 -> Subtract1/1
  Demux/3 -> Subtract2/1
  "thrust "/1 -> [thrust]
  PID Controller/1 -> Subsystem/1(tuned_phi)  "tuned_phi"
  PID Controller1/1 -> Subsystem/2(tuned_theta)  "tuned_theta"
  PID Controller2/1 -> Subsystem/3(tuned_psi)  "tuned_psi"
  Subsystem/1(gamma1) -> w1_square/1
  Subsystem/2(gamma2) -> w2_square/1
  Subsystem/3(gamma3) -> w3_square/1
  Subsystem/4(gamma4) -> w4_square/1

== system correct_sm_circle (1)/Drone Controller/Drone_1 ==
  squares of motor omega in rpm : Inport
  Drone position dynamics : Subsystem
  MMA : Subsystem
  phi_vector : Outport
  x : Outport  Port=2
  y : Outport  Port=3
  z : Outport  Port=4
  wires:
  MMA/2("[Taux;Tauy;Tauz]") -> Drone position dynamics/2(tau_vector)
  MMA/1(Thrust) -> Drone position dynamics/1(thrust)
  Drone position dynamics/1(phi_vector) -> phi_vector/1
  Drone position dynamics/3(y) -> y/1
  Drone position dynamics/4(z) -> z/1
  squares of motor omega in rpm/1 -> MMA/1(w_squares_vector)
  Drone position dynamics/2(x) -> x/1

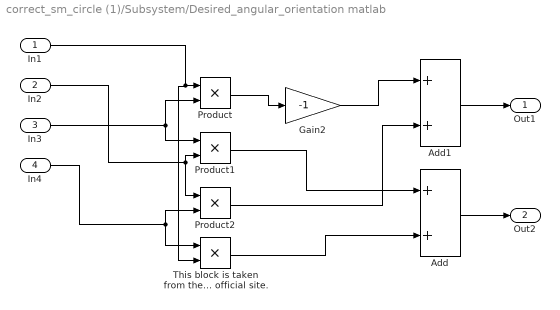
== system correct_sm_circle (1)/Subsystem/Desired_angular_orientation matlab ==
  In1 : Inport
  In2 : Inport  Port=2
  In3 : Inport  Port=3
  In4 : Inport  Port=4
  Add : Sum
  Add1 : Sum
  Gain2 : Gain  Gain=-1
  Product : Product
  Product1 : Product
  Product2 : Product
  This block is taken from the X-rotor quadrotor reference example at Matlab official site. : Product
  Out1 : Outport
  Out2 : Outport  Port=2
  wires:
  Product/1 -> Gain2/1
  Product1/1 -> Add/1
  In2/1 -> Product2/1, Product1/2
  This block is taken from the X-rotor quadrotor reference example at Matlab official site./1 -> Add/2
  In3/1 -> Product1/1, Product/2
  In4/1 -> This block is taken from the X-rotor quadrotor reference example at Matlab official site./1, Product2/2
  Product2/1 -> Add1/2
  Gain2/1 -> Add1/1
  In1/1 -> This block is taken from the X-rotor quadrotor reference example at Matlab official site./2, Product/1
  Add1/1 -> Out1/1
  Add/1 -> Out2/1

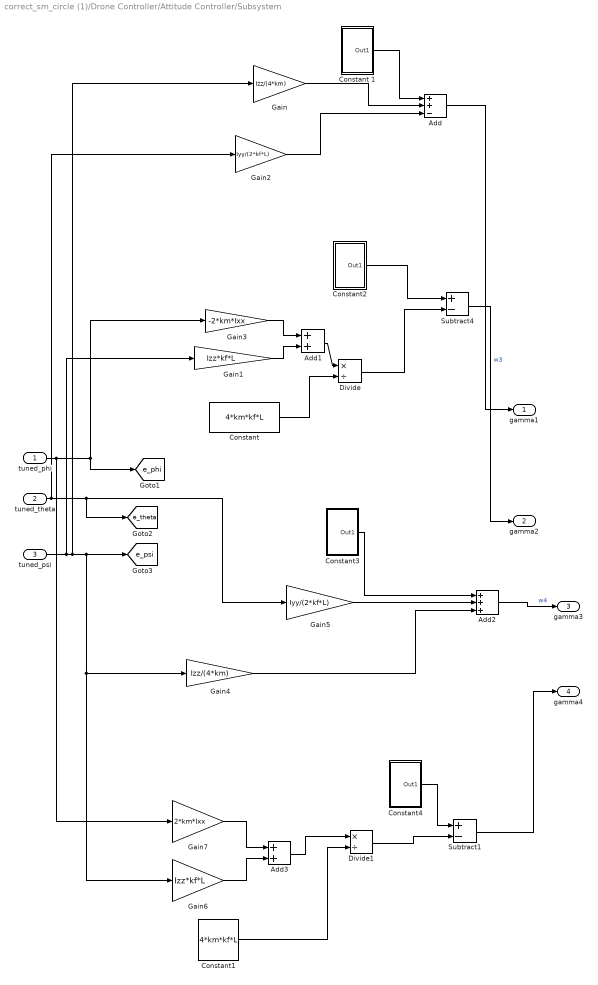
== system correct_sm_circle (1)/Drone Controller/Attitude Controller/Subsystem ==
  tuned_phi : Inport
  tuned_theta : Inport  Port=2
  tuned_psi : Inport  Port=3
  Add : Sum  Inputs=++-
  Add1 : Sum
  Add2 : Sum  Inputs=+++
  Add3 : Sum
  Constant : Constant  Value=4*km*kf*L
  Constant 1 : Subsystem
  Constant1 : Constant  Value=4*km*kf*L
  Constant2 : Subsystem
  Constant3 : Subsystem
  Constant4 : Subsystem
  Divide : Product  Inputs=*/
  Divide1 : Product  Inputs=*/
  Gain : Gain  Gain=Izz/(4*km)
  Gain1 : Gain  Gain=Izz*kf*L
  Gain2 : Gain  Gain=Iyy/(2*kf*L)
  Gain3 : Gain  Gain=-2*km*Ixx
  Gain4 : Gain  Gain=Izz/(4*km)
  Gain5 : Gain  Gain=Iyy/(2*kf*L)
  Gain6 : Gain  Gain=Izz*kf*L
  Gain7 : Gain  Gain=2*km*Ixx
  Subtract1 : Sum  Inputs=+-
  Subtract4 : Sum  Inputs=+-
  gamma1 : Outport
  gamma2 : Outport  Port=2
  gamma3 : Outport  Port=3
  gamma4 : Outport  Port=4
  tag scope: e_phi=global, e_psi=global, e_theta=global
  wires:
  Add/1 -> gamma1/1
  Subtract1/1 -> gamma4/1
  Gain2/1 -> Add/3
  Gain/1 -> Add/2
  Constant 1/1(Out1) -> Add/1
  Constant/1 -> Divide/2
  Add1/1 -> Divide/1
  Divide/1 -> Subtract4/2
  Gain3/1 -> Add1/1
  Subtract4/1 -> gamma2/1  "w3"
  Constant2/1(Out1) -> Subtract4/1
  Gain1/1 -> Add1/2
  Gain4/1 -> Add2/3
  tuned_theta/1 -> [e_theta], Gain5/1, Gain2/1
  Add2/1 -> gamma3/1  "w4"
  Gain5/1 -> Add2/2
  Constant3/1(Out1) -> Add2/1
  tuned_psi/1 -> Gain6/1, Gain4/1, [e_psi], Gain/1, Gain1/1
  Constant1/1 -> Divide1/2
  Constant4/1(Out1) -> Subtract1/1
  Gain6/1 -> Add3/2
  tuned_phi/1 -> Gain3/1, [e_phi], Gain7/1
  Divide1/1 -> Subtract1/2
  Gain7/1 -> Add3/1
  Add3/1 -> Divide1/1

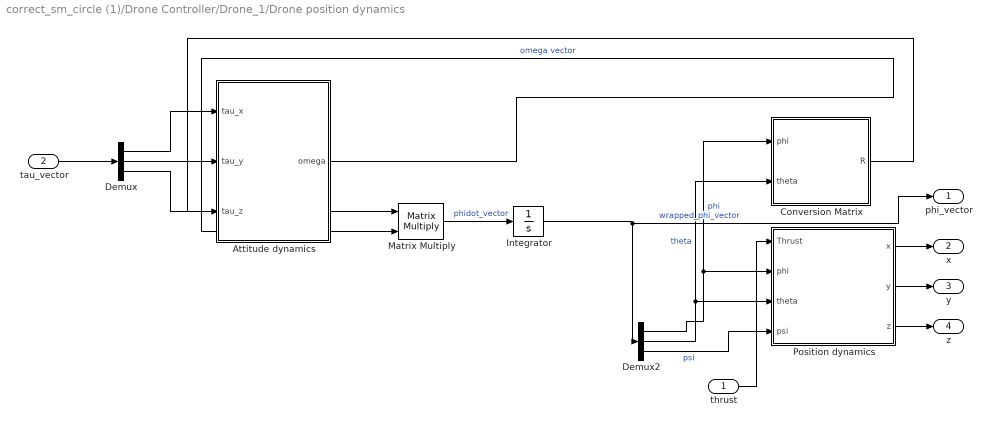
== system correct_sm_circle (1)/Drone Controller/Drone_1/Drone position dynamics ==
  thrust : Inport
  tau_vector : Inport  Port=2
  Attitude dynamics : Subsystem
  Conversion Matrix : MATLAB Function  TreatAsAtomicUnit=on
  Demux : Demux  Outputs=3
  Demux2 : Demux  Outputs=3
  Integrator : Integrator  WrapState=on
  Matrix Multiply : Product  Multiplication=Matrix(*)
  Position dynamics : Subsystem
  phi_vector : Outport
  x : Outport  Port=2
  y : Outport  Port=3
  z : Outport  Port=4
  wires:
  Attitude dynamics/1("omega ") -> Matrix Multiply/2  "omega vector"
  Conversion Matrix/1(R) -> Matrix Multiply/1
  Integrator/1 -> Demux2/1, phi_vector/1  "wrapped_phi_vector"
  Demux2/2 -> Conversion Matrix/2(theta), Position dynamics/3(theta)  "theta"
  Matrix Multiply/1 -> Integrator/1  "phidot_vector"
  Demux2/1 -> Conversion Matrix/1(phi), Position dynamics/2(phi)  "phi"
  Demux2/3 -> Position dynamics/4(psi)  "psi"
  thrust/1 -> Position dynamics/1(Thrust)
  Position dynamics/1(x) -> x/1
  Demux/1 -> Attitude dynamics/1(tau_x)
  Demux/2 -> Attitude dynamics/2(tau_y)
  Demux/3 -> Attitude dynamics/3(tau_z)
  tau_vector/1 -> Demux/1
  Position dynamics/2(y) -> y/1
  Position dynamics/3(z) -> z/1

== system correct_sm_circle (1)/Drone Controller/Drone_1/MMA ==
  w_squares_vector : Inport
  Demux : Demux
  Mux1 : Mux  Inputs=3
  Thrust and Torque Block : Subsystem
  Thrust : Outport
  "[Taux;Tauy;Tauz]" : Outport  Port=2
  wires:
  Demux/4 -> Mux1/3
  Demux/3 -> Mux1/2
  Demux/2 -> Mux1/1
  Mux1/1 -> "[Taux;Tauy;Tauz]"/1
  Demux/1 -> Thrust/1
  w_squares_vector/1 -> Thrust and Torque Block/1(w_squares_vector)
  Thrust and Torque Block/1(Out1) -> Demux/1

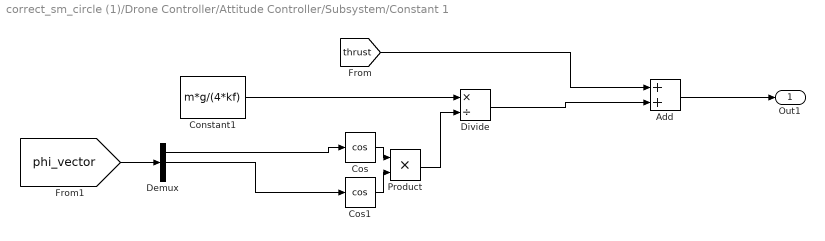
== system correct_sm_circle (1)/Drone Controller/Attitude Controller/Subsystem/Constant 1 ==
  Add : Sum
  Constant1 : Constant  Value=m*g/(4*kf)
  Cos : Trigonometry  Operator=cos
  Cos1 : Trigonometry  Operator=cos
  Demux : Demux  Outputs=3
  Divide : Product  Inputs=*/
  Product : Product
  Out1 : Outport
  wires:
  Add/1 -> Out1/1
  Cos1/1 -> Product/2
  Product/1 -> Divide/2
  Constant1/1 -> Divide/1
  Demux/2 -> Cos1/1
  Demux/1 -> Cos/1
  [phi_vector] -> Demux/1
  Divide/1 -> Add/2
  Cos/1 -> Product/1
  [thrust] -> Add/1

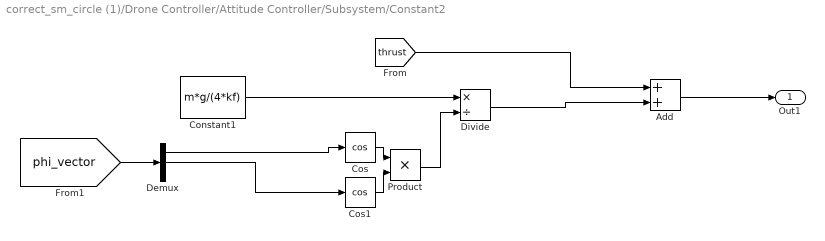
== system correct_sm_circle (1)/Drone Controller/Attitude Controller/Subsystem/Constant2 ==
  Add : Sum
  Constant1 : Constant  Value=m*g/(4*kf)
  Cos : Trigonometry  Operator=cos
  Cos1 : Trigonometry  Operator=cos
  Demux : Demux  Outputs=3
  Divide : Product  Inputs=*/
  Product : Product
  Out1 : Outport
  wires:
  Add/1 -> Out1/1
  Cos1/1 -> Product/2
  Product/1 -> Divide/2
  Constant1/1 -> Divide/1
  Demux/2 -> Cos1/1
  Demux/1 -> Cos/1
  [phi_vector] -> Demux/1
  Divide/1 -> Add/2
  Cos/1 -> Product/1
  [thrust] -> Add/1

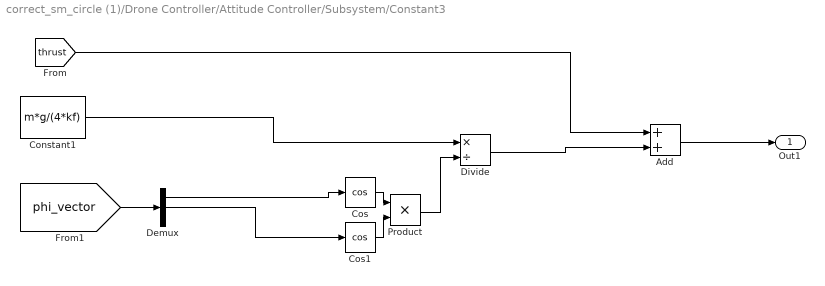
== system correct_sm_circle (1)/Drone Controller/Attitude Controller/Subsystem/Constant3 ==
  Add : Sum
  Constant1 : Constant  Value=m*g/(4*kf)
  Cos : Trigonometry  Operator=cos
  Cos1 : Trigonometry  Operator=cos
  Demux : Demux  Outputs=3
  Divide : Product  Inputs=*/
  Product : Product
  Out1 : Outport
  wires:
  [thrust] -> Add/1
  Cos/1 -> Product/1
  Divide/1 -> Add/2
  [phi_vector] -> Demux/1
  Demux/1 -> Cos/1
  Demux/2 -> Cos1/1
  Constant1/1 -> Divide/1
  Product/1 -> Divide/2
  Cos1/1 -> Product/2
  Add/1 -> Out1/1

== system correct_sm_circle (1)/Drone Controller/Attitude Controller/Subsystem/Constant4 ==
  Add : Sum
  Constant1 : Constant  Value=m*g/(4*kf)
  Cos : Trigonometry  Operator=cos
  Cos1 : Trigonometry  Operator=cos
  Demux : Demux  Outputs=3
  Divide : Product  Inputs=*/
  Product : Product
  Out1 : Outport
  wires:
  Add/1 -> Out1/1
  Cos1/1 -> Product/2
  Product/1 -> Divide/2
  Constant1/1 -> Divide/1
  Demux/2 -> Cos1/1
  Demux/1 -> Cos/1
  [phi_vector] -> Demux/1
  Divide/1 -> Add/2
  Cos/1 -> Product/1
  [thrust] -> Add/1

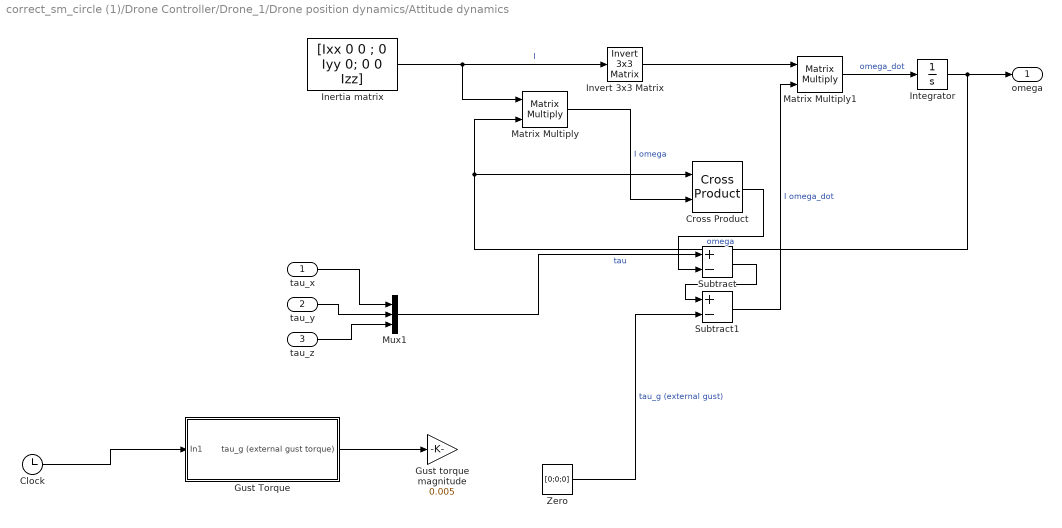
== system correct_sm_circle (1)/Drone Controller/Drone_1/Drone position dynamics/Attitude dynamics ==
  tau_x : Inport
  tau_y : Inport  Port=2
  tau_z : Inport  Port=3
  Clock : Clock
  Cross Product : matrix_library/Cross Product
  Gust Torque : Subsystem
  Gust torque magnitude : Gain  Gain=0.005
  Inertia matrix : Constant  Value=[Ixx 0 0 ; 0 Iyy 0; 0 0 Izz]
  Integrator : Integrator  WrapState=on
  Invert 3x3 Matrix : aerolibutil/Invert  3x3 Matrix
  Matrix Multiply : Product  Multiplication=Matrix(*)
  Matrix Multiply1 : Product  Multiplication=Matrix(*)
  Mux1 : Mux  Inputs=3
  Subtract : Sum  Inputs=+-
  Subtract1 : Sum  Inputs=+-
  Zero : Constant  Value=[0;0;0]  OutDataTypeStr=Inherit: Inherit via back propagation
  "omega " : Outport
  wires:
  Integrator/1 -> "omega "/1, Matrix Multiply/2, Cross Product/1  "omega"
  Matrix Multiply/1 -> Cross Product/2  "I omega"
  Inertia matrix/1 -> Invert 3x3 Matrix/1, Matrix Multiply/1  "I"
  Zero/1 -> Subtract1/2  "tau_g (external gust)"
  Subtract/1 -> Subtract1/1
  Cross Product/1 -> Subtract/2
  Mux1/1 -> Subtract/1  "tau"
  tau_y/1 -> Mux1/2
  tau_z/1 -> Mux1/3
  tau_x/1 -> Mux1/1
  Subtract1/1 -> Matrix Multiply1/2  "I omega_dot"
  Invert 3x3 Matrix/1 -> Matrix Multiply1/1
  Matrix Multiply1/1 -> Integrator/1  "omega_dot"
  Clock/1 -> Gust Torque/1(In1)
  Gust Torque/1(tau_g (external gust torque)) -> Gust torque magnitude/1

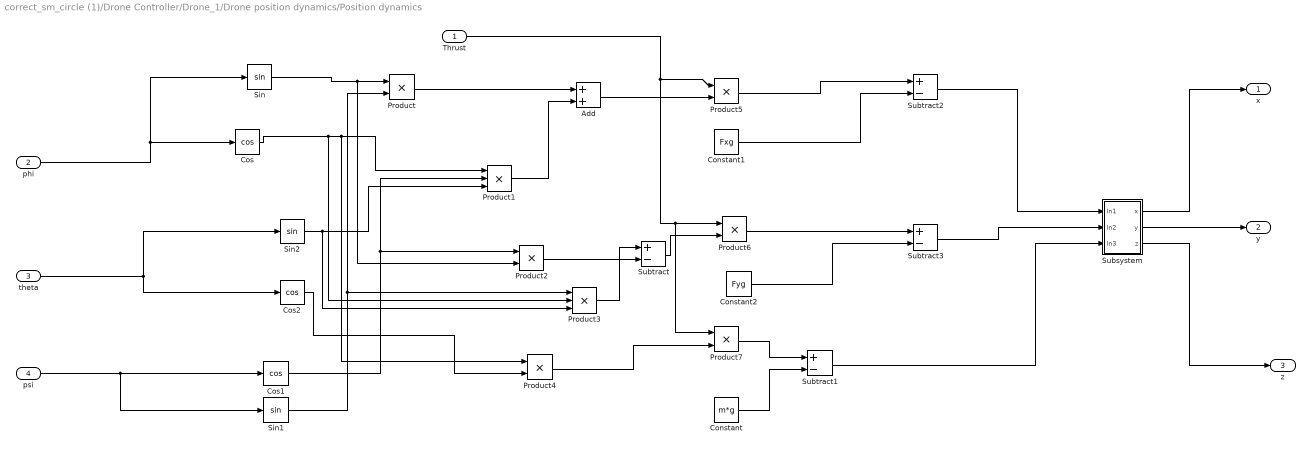
== system correct_sm_circle (1)/Drone Controller/Drone_1/Drone position dynamics/Position dynamics ==
  Thrust : Inport
  phi : Inport  Port=2
  theta : Inport  Port=3
  psi : Inport  Port=4
  Add : Sum
  Constant : Constant  Value=m*g
  Constant1 : Constant  Value=Fxg
  Constant2 : Constant  Value=Fyg
  Cos : Trigonometry  Operator=cos
  Cos1 : Trigonometry  Operator=cos
  Cos2 : Trigonometry  Operator=cos
  Product{,2,4..7} (6 alike) : Product
  Product1 : Product  Inputs=3
  Product3 : Product  Inputs=3
  Sin : Trigonometry
  Sin1 : Trigonometry
  Sin2 : Trigonometry
  Subsystem : Subsystem
  Subtract{,1..3} (4 alike) : Sum  Inputs=+-
  x : Outport
  y : Outport  Port=2
  z : Outport  Port=3
  wires:
  Product7/1 -> Subtract1/1
  Product/1 -> Add/1
  phi/1 -> Sin/1, Cos/1
  Product1/1 -> Add/2
  Cos/1 -> Product3/2, Product4/1, Product1/1
  Sin1/1 -> Product3/1, Product/2
  Product6/1 -> Subtract3/1
  Sin/1 -> Product2/2, Product/1
  Product5/1 -> Subtract2/1
  Thrust/1 -> Product7/1, Product6/1, Product5/1
  psi/1 -> Sin1/1, Cos1/1
  Cos2/1 -> Product4/2
  Product4/1 -> Product7/2
  Cos1/1 -> Product2/1, Product1/2
  Product3/1 -> Subtract/1
  Sin2/1 -> Product3/3, Product1/3
  Product2/1 -> Subtract/2
  Subtract/1 -> Product6/2
  Constant1/1 -> Subtract2/2
  theta/1 -> Cos2/1, Sin2/1
  Constant/1 -> Subtract1/2
  Add/1 -> Product5/2
  Constant2/1 -> Subtract3/2
  Subtract2/1 -> Subsystem/1(In1)
  Subtract3/1 -> Subsystem/2(In2)
  Subtract1/1 -> Subsystem/3(In3)
  Subsystem/1(x) -> x/1
  Subsystem/2(y) -> y/1
  Subsystem/3(z) -> z/1

== system correct_sm_circle (1)/Drone Controller/Drone_1/MMA/Thrust and Torque Block ==
  w_squares_vector : Inport
  Matrix Multiply : Product  Multiplication=Matrix(*)
  Matrix Provided in Exam with added thrust block : Constant  Value=[kf kf kf kf; 0 kf*L 0 -kf*L; -kf*L 0 kf*L 0; km -km km -km]
  Out1 : Outport
  wires:
  w_squares_vector/1 -> Matrix Multiply/2
  Matrix Multiply/1 -> Out1/1
  Matrix Provided in Exam with added thrust block/1 -> Matrix Multiply/1

== system correct_sm_circle (1)/Drone Controller/Drone_1/Drone position dynamics/Attitude dynamics/Gust Torque ==
  In1 : Inport
  Cos : Trigonometry  Operator=cos
  Gain : Gain  Gain=2
  Mux2 : Mux  Inputs=3
  Sin : Trigonometry
  tau_g (external gust torque) : Outport
  wires:
  Mux2/1 -> tau_g (external gust torque)/1  "tau_g (external gust torque)"
  In1/1 -> Cos/1, Sin/1
  Gain/1 -> Mux2/3
  Sin/1 -> Gain/1, Mux2/2
  Cos/1 -> Mux2/1

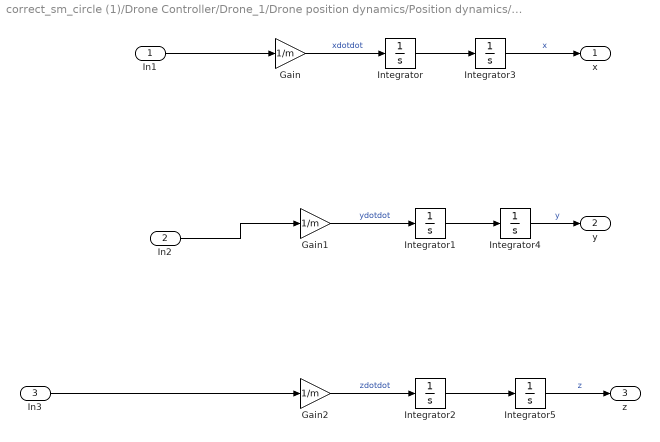
== system correct_sm_circle (1)/Drone Controller/Drone_1/Drone position dynamics/Position dynamics/Subsystem ==
  In1 : Inport
  In2 : Inport  Port=2
  In3 : Inport  Port=3
  Gain : Gain  Gain=1/m
  Gain1 : Gain  Gain=1/m
  Gain2 : Gain  Gain=1/m
  Integrator{,1..4} (5 alike) : Integrator
  Integrator5 : Integrator  LimitOutput=on  LowerSaturationLimit=0
  x : Outport
  y : Outport  Port=2
  z : Outport  Port=3
  wires:
  Integrator4/1 -> y/1  "y"
  In2/1 -> Gain1/1
  Gain/1 -> Integrator/1  "xdotdot"
  Integrator/1 -> Integrator3/1
  Integrator1/1 -> Integrator4/1
  Gain1/1 -> Integrator1/1  "ydotdot"
  Integrator2/1 -> Integrator5/1
  Gain2/1 -> Integrator2/1  "zdotdot"
  Integrator5/1 -> z/1  "z"
  Integrator3/1 -> x/1  "x"
  In1/1 -> Gain/1
  In3/1 -> Gain2/1

== matlab function correct_sm_circle (1)/Drone Controller/Drone_1/Drone position dynamics/Conversion Matrix ==
  data: phi input; R output; theta input
function R = fcn(phi,theta)
R = [1 0 -sin(theta) ; 0 cos(phi) cos(theta)*sin(phi) ; 0 -sin(phi) cos(theta)*cos(phi)] ;
